simulink model "Full_model"  (R2021a)
settings: Solver=FixedStepAuto  StartTime=0  StopTime=50  FixedStep=0.001  RelTol=1e-3
settings Model: Creator=antho  LastModifiedBy=antho

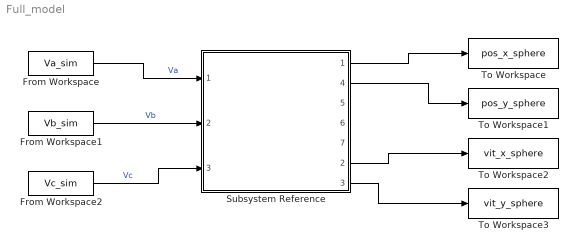
== system Full_model ==
  From Workspace : FromWorkspace  VariableName=Va_sim
  From Workspace1 : FromWorkspace  VariableName=Vb_sim
  From Workspace2 : FromWorkspace  VariableName=Vc_sim
  Subsystem Reference : Subsystem  ReferencedSubsystem=subsys_Full_Model_NL
      settings: PortSchema="{\"entries\":[{\"content\":{\"sides\":[{\"content\":{\"connectorIds\":[\"In1\",\"In2\",\"In3\"]},\"type\":\"ConnectorPlacement.EquallySpacedRectSide\",\"uuid\":\"4a718a88-38a5-47c8-a698-203ac9a4fd64\"},{\"content\":{\"connectorIds\":[\"Out1\",\"Out4\",\"Out5\",\"Out6\",\"Out7\",\"Out2\",\"Out3\"],\"side\":\"RIGHT\"},\"type\":\"ConnectorPlacement.EquallySpacedRectSide\",\"uuid\":\"d98c962f-ab29-42d9-aa34-79f3659eb7f8\"},{\"content\":{\"connectorIds\":[],\"side\":\"TOP\"},\"type\":\"ConnectorPlacement.EquallySpacedRectSide\",\"uuid\":\"c7db5e38-732b-4374-a404-09d1c22c3b00\"}]},\"type\":\"ConnectorPlacement.EquallySpacedConnector\",\"uuid\":\"a7b40d99-f7cd-4400-8491-dba9e8ad6d23\"}],\"packageUris\":[\"http://schema.mathworks.com/mf0/Connector/R2020b\"],\"version\":\"1.0\"}"
  To Workspace : ToWorkspace  VariableName=pos_x_sphere  SaveFormat=Timeseries  SampleTime=-1
  To Workspace1 : ToWorkspace  VariableName=pos_y_sphere  SaveFormat=Timeseries  SampleTime=-1
  To Workspace2 : ToWorkspace  VariableName=vit_x_sphere  SaveFormat=Timeseries  SampleTime=-1
  To Workspace3 : ToWorkspace  VariableName=vit_y_sphere  SaveFormat=Timeseries  SampleTime=-1
  wires:
  From Workspace/1 -> Subsystem Reference/1  "Va"
  From Workspace1/1 -> Subsystem Reference/2  "Vb"
  From Workspace2/1 -> Subsystem Reference/3  "Vc"
  Subsystem Reference/4 -> To Workspace1/1
  Subsystem Reference/1 -> To Workspace/1
  Subsystem Reference/2 -> To Workspace2/1
  Subsystem Reference/3 -> To Workspace3/1
